simulink model "UDP_2018b"  (R2021b)
settings: Solver=FixedStepAuto  StartTime=0.0  StopTime=inf  FixedStep=0.01  RelTol=1e-3
undefined symbols (not defined in the file): Angle, Axis, magnitude, R_threshold, theta1
libraries: dspstat3 x3, dspnetwork x2, simulink_extras x1, robotcorelib x1
settings Model: Creator=OKADA  LastModifiedBy=村尾研究室
settings SolverCC: AlgebraicLoopSolver=TrustRegion
settings DataIOCC: ReturnWorkspaceOutputs=off
settings DebuggingCC: SFMachineParentedDataDiag=warning  ArithmeticOperatorsInVariantConditions=warning
settings SFSimCC: CustomCodeUndefinedFunction=UseInterfaceOnly
settings RTWCC: DLArmComputeVersion=20.02.1

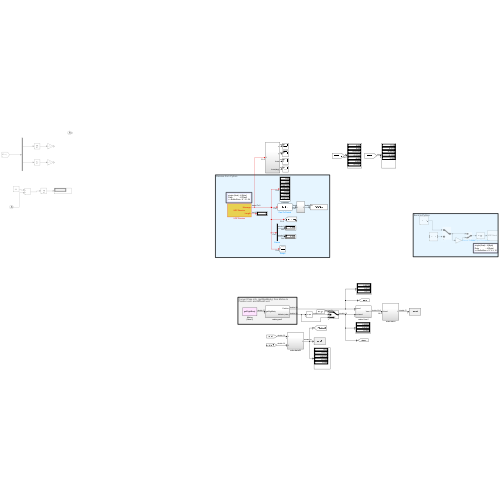
[thumbnail: Simulink's stored preview of the top-level diagram]
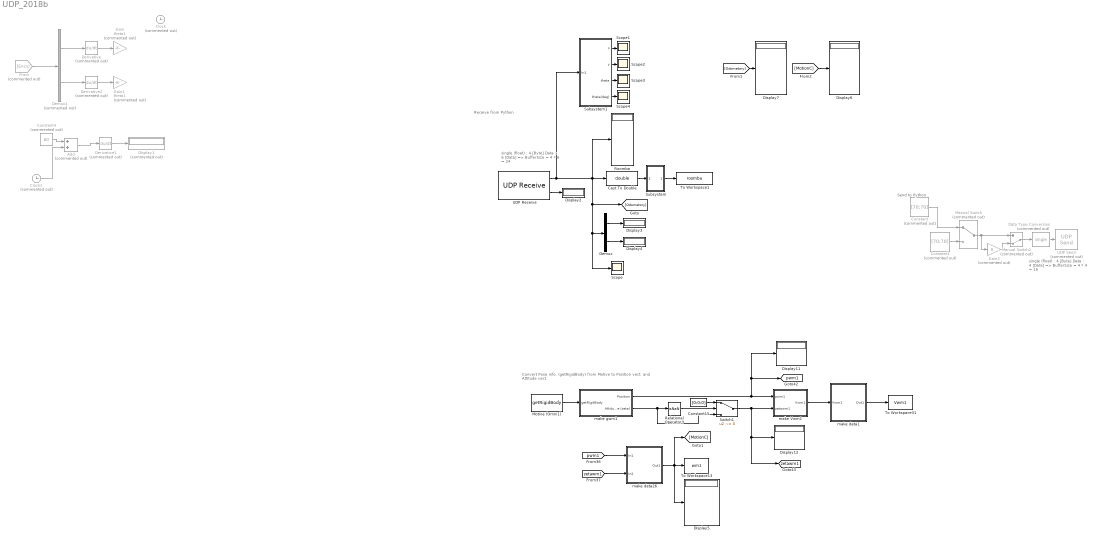
== system UDP_2018b ==
  note: Send to Python
  note: Receive from Python
  note: single (float) : 4 [Byte]
      | Data             : 6 [Data]
      | => BufferSize = 4 * 6 = 24
  note: single (float) : 4 [Byte]
      | Data             : 4 [Data]
      | => BufferSize = 4 * 4 = 16
  note: Convert Pose info. (getRigidBody) from Motive to
      | Position vect. and Attitude vect.
  Add : Sum  Commented=on
  Cast To Double : DataTypeConversion  OutDataTypeStr=double
  Clock : Clock  Commented=on
  Clock1 : Clock  Commented=on
  Constant : Constant  Commented=on  Value=[70;70]
  Constant1 : Constant  Commented=on  Value=[70;70]
  Constant15 : Constant  Value=[0;0;0]
  Constant4 : Constant  Commented=on  Value=60
  Data Type Conversion : DataTypeConversion  Commented=on  OutDataTypeStr=single
  Demux : Demux  Outputs=2
  Demux1 : Demux  Commented=on  Outputs=2
  Derivative : Derivative  Commented=on
  Derivative1 : Derivative  Commented=on
  Derivative2 : Derivative  Commented=on
  Display1 : Display  Commented=on
  Display{2..7,11..12} (8 alike) : Display
  From : From  Commented=on  GotoTag=Encs
  Gain : Gain  Commented=on  Gain=theta1
  Gain1 : Gain  Commented=on  Gain=theta1
  Gain3 : Gain  Commented=on  Gain=0
  Manual Switch : ManualSwitch  Commented=on
  Manual Switch2 : ManualSwitch  Commented=on  CurrentSetting=0
  Motive (Omni1) : M-S-Function  FunctionName=getRigidBody  Parameters=1
  Relational Operator3 : RelationalOperator  Operator=isNaN  OutDataTypeStr=boolean  RndMeth=Simplest
  Roomba : Display
  Scope{,1..4} (5 alike) : Scope
  Subsystem : Subsystem
  Subsystem1 : Subsystem
  Switch1 : Switch  Criteria=u2 ~= 0
  To Workspace1 : ToWorkspace  VariableName=roomba  SaveFormat=Structure With Time  SampleTime=-1
  To Workspace13 : ToWorkspace  VariableName=wm1  SaveFormat=Structure With Time  SampleTime=-1
  To Workspace31 : ToWorkspace  VariableName=Vwm1  SaveFormat=Structure With Time  SampleTime=-1
  UDP Receive : dspnetwork/UDP Receive  localURL='0.0.0.0'  localPort=4000  remoteURL='127.0.0.1'  remotePort=-1  recvBufferSize=28  dims=7  signalDatatype=single  isComplex=off  isVarSize=off  showBlockingTime=off  blockingTime=0  sampletime=0.01  blockPlatform=[]
  UDP Send : dspnetwork/UDP Send  Commented=on  remoteURL='127.0.0.1'  remotePort=8000  localURL='0.0.0.0'  localPortSource=Automatically determine  localPort=-1  sendBufferSize=8192  sampletime=-1  blockPlatform=[]  separateLengthPort=0
  make Vwm1 : Subsystem
  make data1 : Subsystem
  make data26 : Subsystem
  make gwm1 : Subsystem
  tag scope: pwm1=global, zetawm1=global
  wires:
  UDP Receive/2 -> Display2/1
  UDP Receive/1 -> Subsystem1/1(In1), Cast To Double/1, Roomba/1, [Odometory], Scope/1, Demux/1
  Demux/1 -> Display3/1
  Demux/2 -> Display4/1
  Manual Switch/1 -> Gain3/1, Manual Switch2/1
  Data Type Conversion/1 -> UDP Send/1
  Constant/1 -> Manual Switch/1
  Gain3/1 -> Manual Switch2/2
  Constant4/1 -> Add/1
  Add/1 -> Derivative1/1
  Clock1/1 -> Add/2
  Derivative1/1 -> Display1/1
  From/1 -> Demux1/1
  Demux1/1 -> Derivative/1
  Demux1/2 -> Derivative2/1
  Derivative/1 -> Gain/1
  Derivative2/1 -> Gain1/1
  Motive (Omni1)/1 -> make gwm1/1(getRigitBody)
  Relational Operator3/1 -> Switch1/2
  make data1/1(Out1) -> To Workspace31/1
  make gwm1/1(Position) -> make Vwm1/1(pwm1), [pwm1], Display11/1
  make data26/1(Out1) -> [MotionC], To Workspace13/1, Display5/1
  [zetawm1] -> make data26/2(In2)
  make Vwm1/1(Vwm1) -> make data1/1(Vwm1)
  [pwm1] -> make data26/1(In1)
  Switch1/1 -> make Vwm1/2(zetawm1), [zetawm1], Display12/1
  Constant15/1 -> Switch1/1
  make gwm1/2(Attitude (zeta)) -> Switch1/3, Relational Operator3/1
  Cast To Double/1 -> Subsystem/1(In1)
  Subsystem/1(Out1) -> To Workspace1/1
  Manual Switch2/1 -> Data Type Conversion/1
  Constant1/1 -> Manual Switch/2
  Subsystem1/1(x) -> Scope1/1
  Subsystem1/2(y) -> Scope2/1
  Subsystem1/3(theta) -> Scope3/1
  Subsystem1/4(theta(deg)) -> Scope4/1
  [MotionC] -> Display6/1
  [Odometory] -> Display7/1

== system UDP_2018b/Subsystem ==
  In1 : Inport
  Clock2 : Clock
  Demux3 : Demux  Outputs=7
  Mux2 : Mux  Inputs=8
  Out1 : Outport
  wires:
  Demux3/6 -> Mux2/7
  Demux3/1 -> Mux2/2
  Mux2/1 -> Out1/1
  Demux3/5 -> Mux2/6
  Demux3/4 -> Mux2/5
  Demux3/7 -> Mux2/8
  In1/1 -> Demux3/1
  Demux3/3 -> Mux2/4
  Clock2/1 -> Mux2/1
  Demux3/2 -> Mux2/3

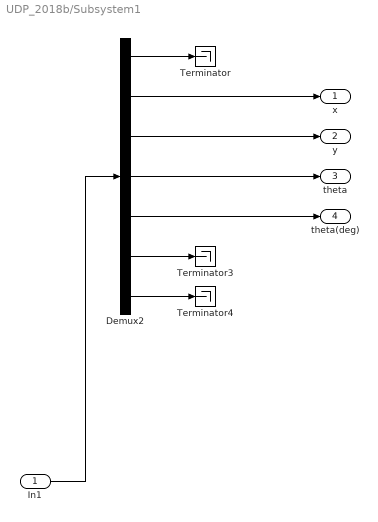
== system UDP_2018b/Subsystem1 ==
  In1 : Inport
  Demux2 : Demux  Outputs=7
  Terminator : Terminator
  Terminator3 : Terminator
  Terminator4 : Terminator
  x : Outport
  y : Outport  Port=2
  theta : Outport  Port=3
  theta(deg) : Outport  Port=4
  wires:
  Demux2/7 -> Terminator4/1
  Demux2/5 -> theta(deg)/1
  Demux2/4 -> theta/1
  Demux2/6 -> Terminator3/1
  Demux2/2 -> x/1
  In1/1 -> Demux2/1
  Demux2/1 -> Terminator/1
  Demux2/3 -> y/1

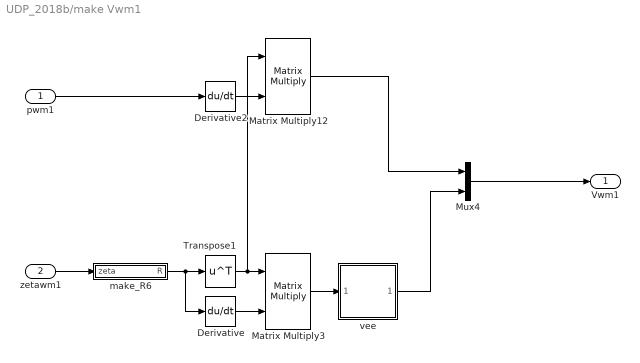
== system UDP_2018b/make Vwm1 ==
  pwm1 : Inport
  zetawm1 : Inport  Port=2
  Derivative : Derivative
  Derivative2 : Derivative
  Matrix Multiply12 : Product  Multiplication=Matrix(*)
  Matrix Multiply3 : Product  Multiplication=Matrix(*)
  Mux4 : Mux  Inputs=2
  Transpose1 : Math  Operator=transpose  SaturateOnIntegerOverflow=on
  make_R6 : Subsystem
  vee : Subsystem
  Vwm1 : Outport
  wires:
  Derivative2/1 -> Matrix Multiply12/2
  Matrix Multiply3/1 -> vee/1("[3*3]")
  Derivative/1 -> Matrix Multiply3/2
  make_R6/1(R) -> Derivative/1, Transpose1/1
  vee/1("[3*1]") -> Mux4/2
  Transpose1/1 -> Matrix Multiply12/1, Matrix Multiply3/1
  zetawm1/1 -> make_R6/1(zeta)
  Matrix Multiply12/1 -> Mux4/1
  pwm1/1 -> Derivative2/1
  Mux4/1 -> Vwm1/1

== system UDP_2018b/make data1 ==
  Vwm1 : Inport
  Clock1 : Clock
  Demux4 : Demux  Outputs=6
      settings: DisplayOption=none
  Mux2 : Mux  Inputs=7
  Out1 : Outport
  wires:
  Demux4/4 -> Mux2/5
  Demux4/5 -> Mux2/6
  Demux4/6 -> Mux2/7
  Demux4/3 -> Mux2/4
  Demux4/2 -> Mux2/3
  Demux4/1 -> Mux2/2
  Vwm1/1 -> Demux4/1
  Mux2/1 -> Out1/1
  Clock1/1 -> Mux2/1

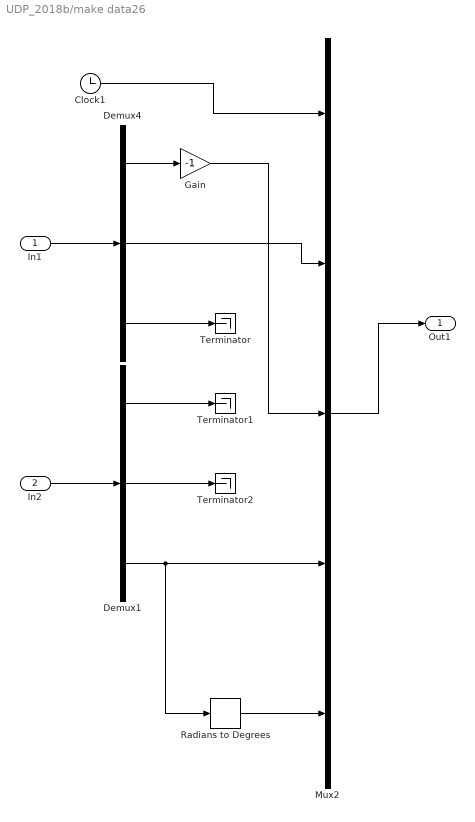
== system UDP_2018b/make data26 ==
  In1 : Inport
  In2 : Inport  Port=2
  Clock1 : Clock
  Demux1 : Demux  Outputs=3
      settings: DisplayOption=none
  Demux4 : Demux  Outputs=3
      settings: DisplayOption=none
  Gain : Gain  Gain=-1
  Mux2 : Mux  Inputs=5
  Radians to Degrees : simulink_extras/Transformations/Radians to Degrees
  Terminator : Terminator
  Terminator1 : Terminator
  Terminator2 : Terminator
  Out1 : Outport
  wires:
  Gain/1 -> Mux2/3
  Radians to Degrees/1 -> Mux2/5
  Demux1/2 -> Terminator2/1
  Demux1/1 -> Terminator1/1
  Demux4/3 -> Terminator/1
  In2/1 -> Demux1/1
  Demux1/3 -> Mux2/4, Radians to Degrees/1
  Clock1/1 -> Mux2/1
  Mux2/1 -> Out1/1
  In1/1 -> Demux4/1
  Demux4/1 -> Gain/1
  Demux4/2 -> Mux2/2

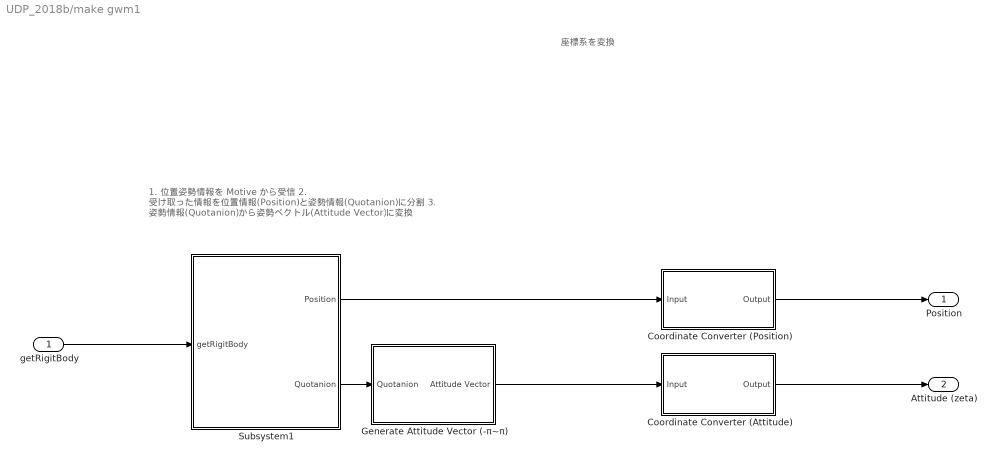
== system UDP_2018b/make gwm1 ==
  note: 1. 位置姿勢情報を Motive から受信
      | 2. 受け取った情報を位置情報(Position)と姿勢情報(Quotanion)に分割
      | 3. 姿勢情報(Quotanion)から姿勢ベクトル(Attitude Vector)に変換
  note: 座標系を変換
  getRigitBody : Inport
  Coordinate Converter (Attitude) : Subsystem
  Coordinate Converter (Position) : Subsystem
  Generate Attitude Vector (-π~π) : Subsystem
  Subsystem1 : Subsystem
  Position : Outport  VectorParamsAs1DForOutWhenUnconnected=off
  Attitude (zeta) : Outport  Port=2  VectorParamsAs1DForOutWhenUnconnected=off
  wires:
  Coordinate Converter (Attitude)/1(Output) -> Attitude (zeta)/1
  Coordinate Converter (Position)/1(Output) -> Position/1
  Subsystem1/1(Position) -> Coordinate Converter (Position)/1(Input)
  Generate Attitude Vector (-π~π)/1(Attitude Vector) -> Coordinate Converter (Attitude)/1(Input)
  getRigitBody/1 -> Subsystem1/1(getRigitBody)
  Subsystem1/2(Quotanion) -> Generate Attitude Vector (-π~π)/1(Quotanion)

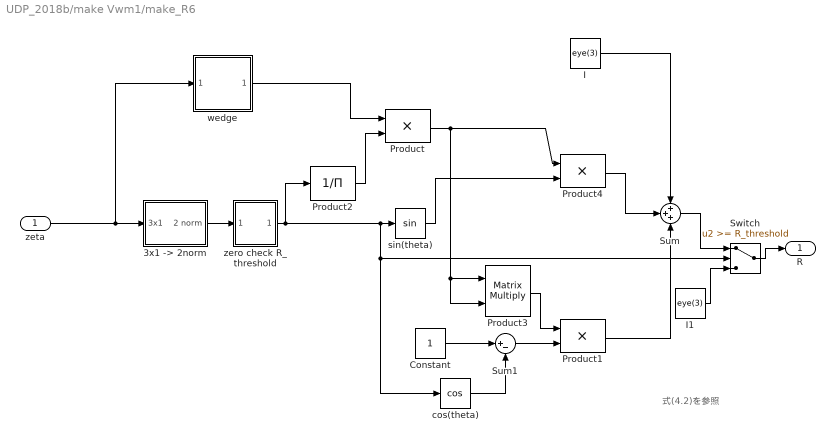
== system UDP_2018b/make Vwm1/make_R6 ==
  note: 式(4.2)を参照
  zeta : Inport
  "3x1 -> 2norm" : Subsystem
  Constant : Constant
  I : Constant  Value=eye(3)  VectorParams1D=off
  I1 : Constant  Value=eye(3)  VectorParams1D=off
  Product : Product  InputSameDT=on  SaturateOnIntegerOverflow=on  OutDataTypeStr=Inherit: Same as first input
  Product1 : Product  InputSameDT=on  SaturateOnIntegerOverflow=on  OutDataTypeStr=Inherit: Same as first input
  Product2 : Product  Inputs=/  InputSameDT=on  SaturateOnIntegerOverflow=on  OutDataTypeStr=Inherit: Same as first input
  Product3 : Product  Multiplication=Matrix(*)  InputSameDT=on  SaturateOnIntegerOverflow=on  OutDataTypeStr=Inherit: Same as first input
  Product4 : Product  InputSameDT=on  SaturateOnIntegerOverflow=on  OutDataTypeStr=Inherit: Same as first input
  Sum : Sum  Inputs=+++  InputSameDT=on  SaturateOnIntegerOverflow=on  OutDataTypeStr=Inherit: Same as first input
  Sum1 : Sum  Inputs=|+-  InputSameDT=on  SaturateOnIntegerOverflow=on  OutDataTypeStr=Inherit: Same as first input
  Switch : Switch  Threshold=R_threshold  SaturateOnIntegerOverflow=on  InputSameDT=on
  cos(theta) : Trigonometry  Operator=cos
  sin(theta) : Trigonometry
  wedge : Subsystem
  zero check R_threshold : Subsystem
  R : Outport  VectorParamsAs1DForOutWhenUnconnected=off
  wires:
  Product4/1 -> Sum/2
  Product1/1 -> Sum/3
  Sum1/1 -> Product1/2
  cos(theta)/1 -> Sum1/2
  Constant/1 -> Sum1/1
  I/1 -> Sum/1
  sin(theta)/1 -> Product4/2
  Sum/1 -> Switch/1
  I1/1 -> Switch/3
  Switch/1 -> R/1
  "3x1 -> 2norm"/1(2 norm) -> zero check R_threshold/1(In1)
  Product/1 -> Product4/1, Product3/1, Product3/2
  wedge/1("[3x3]") -> Product/1
  zero check R_threshold/1(Out1) -> Product2/1, sin(theta)/1, Switch/2, cos(theta)/1
  Product2/1 -> Product/2
  zeta/1 -> "3x1 -> 2norm"/1(3x1), wedge/1("[3x1]")
  Product3/1 -> Product1/1

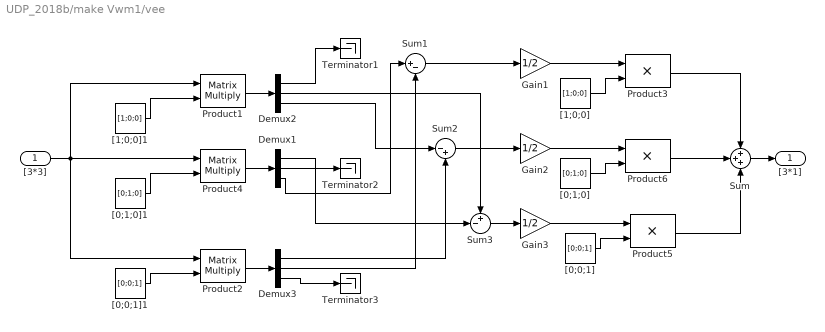
== system UDP_2018b/make Vwm1/vee ==
  "[3*3]" : Inport
  Demux1 : Demux  Outputs=3
      settings: DisplayOption=none
  Demux2 : Demux  Outputs=3
      settings: DisplayOption=none
  Demux3 : Demux  Outputs=3
      settings: DisplayOption=none
  Gain1 : Gain  Gain=1/2  SaturateOnIntegerOverflow=on  OutDataTypeStr=Inherit: Same as input  ParamDataTypeStr=Inherit: Same as input
  Gain2 : Gain  Gain=1/2  SaturateOnIntegerOverflow=on  OutDataTypeStr=Inherit: Same as input  ParamDataTypeStr=Inherit: Same as input
  Gain3 : Gain  Gain=1/2  SaturateOnIntegerOverflow=on  OutDataTypeStr=Inherit: Same as input  ParamDataTypeStr=Inherit: Same as input
  Product1 : Product  Multiplication=Matrix(*)  InputSameDT=on  SaturateOnIntegerOverflow=on  OutDataTypeStr=Inherit: Same as first input
  Product2 : Product  Multiplication=Matrix(*)  InputSameDT=on  SaturateOnIntegerOverflow=on  OutDataTypeStr=Inherit: Same as first input
  Product3 : Product  InputSameDT=on  SaturateOnIntegerOverflow=on  OutDataTypeStr=Inherit: Same as first input
  Product4 : Product  Multiplication=Matrix(*)  InputSameDT=on  SaturateOnIntegerOverflow=on  OutDataTypeStr=Inherit: Same as first input
  Product5 : Product  InputSameDT=on  SaturateOnIntegerOverflow=on  OutDataTypeStr=Inherit: Same as first input
  Product6 : Product  InputSameDT=on  SaturateOnIntegerOverflow=on  OutDataTypeStr=Inherit: Same as first input
  Sum : Sum  Inputs=+++  InputSameDT=on  SaturateOnIntegerOverflow=on  OutDataTypeStr=Inherit: Same as first input
  Sum1 : Sum  Inputs=|+-  InputSameDT=on  SaturateOnIntegerOverflow=on  OutDataTypeStr=Inherit: Same as first input
  Sum2 : Sum  Inputs=|-+  InputSameDT=on  SaturateOnIntegerOverflow=on  OutDataTypeStr=Inherit: Same as first input
  Sum3 : Sum  Inputs=+-|  InputSameDT=on  SaturateOnIntegerOverflow=on  OutDataTypeStr=Inherit: Same as first input
  Terminator1 : Terminator
  Terminator2 : Terminator
  Terminator3 : Terminator
  "[0;0;1]" : Constant  Value=[0;0;1]  VectorParams1D=off
  "[0;0;1]1" : Constant  Value=[0;0;1]  VectorParams1D=off
  "[0;1;0]" : Constant  Value=[0;1;0]  VectorParams1D=off
  "[0;1;0]1" : Constant  Value=[0;1;0]  VectorParams1D=off
  "[1;0;0]" : Constant  Value=[1;0;0]  VectorParams1D=off
  "[1;0;0]1" : Constant  Value=[1;0;0]  VectorParams1D=off
  "[3*1]" : Outport  VectorParamsAs1DForOutWhenUnconnected=off
  wires:
  "[3*3]"/1 -> Product2/1, Product1/1, Product4/1
  "[0;1;0]1"/1 -> Product4/2
  Product4/1 -> Demux1/1
  Demux1/2 -> Terminator2/1
  Demux1/3 -> Sum1/1
  "[1;0;0]1"/1 -> Product1/2
  Product1/1 -> Demux2/1
  Demux2/1 -> Terminator1/1
  "[0;0;1]1"/1 -> Product2/2
  Product2/1 -> Demux3/1
  Demux3/3 -> Terminator3/1
  Demux3/1 -> Sum2/2
  "[1;0;0]"/1 -> Product3/2
  "[0;1;0]"/1 -> Product6/2
  "[0;0;1]"/1 -> Product5/2
  Product6/1 -> Sum/2
  Product5/1 -> Sum/3
  Product3/1 -> Sum/1
  Sum/1 -> "[3*1]"/1
  Sum1/1 -> Gain1/1
  Gain1/1 -> Product3/1
  Demux3/2 -> Sum1/2
  Gain2/1 -> Product6/1
  Gain3/1 -> Product5/1
  Demux2/3 -> Sum2/1
  Sum2/1 -> Gain2/1
  Sum3/1 -> Gain3/1
  Demux2/2 -> Sum3/1
  Demux1/1 -> Sum3/2

== system UDP_2018b/make gwm1/Coordinate Converter (Attitude) ==
  Input : Inport
  Demux : Demux  Outputs=3
  Mux : Mux  Inputs=3
  Output : Outport  VectorParamsAs1DForOutWhenUnconnected=off
  wires:
  Demux/3 -> Mux/1
  Demux/1 -> Mux/2
  Demux/2 -> Mux/3
  Mux/1 -> Output/1
  Input/1 -> Demux/1

== system UDP_2018b/make gwm1/Coordinate Converter (Position) ==
  Input : Inport
  Demux : Demux  Outputs=3
  Mux : Mux  Inputs=3
  Output : Outport  VectorParamsAs1DForOutWhenUnconnected=off
  wires:
  Demux/3 -> Mux/1
  Demux/1 -> Mux/2
  Demux/2 -> Mux/3
  Mux/1 -> Output/1
  Input/1 -> Demux/1

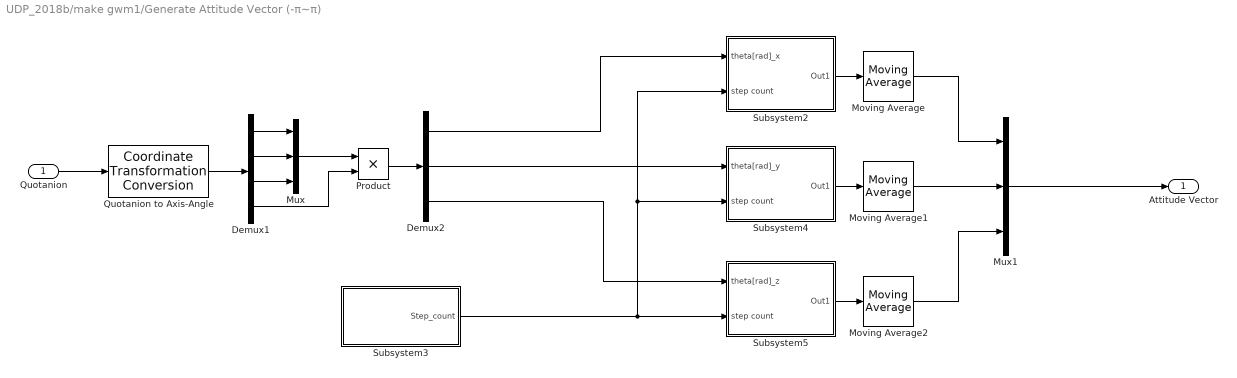
== system UDP_2018b/make gwm1/Generate Attitude Vector (-π~π) ==
  Quotanion : Inport
  Demux1 : Demux
  Demux2 : Demux  Outputs=3
  Moving Average : dspstat3/Moving Average  Method=Sliding window  ForgettingFactorPort=off  SpecifyWindowLength=on  WindowLength=10  ForgettingFactor=0.9  SimulateUsing=Code generation
  Moving Average1 : dspstat3/Moving Average  Method=Sliding window  ForgettingFactorPort=off  SpecifyWindowLength=on  WindowLength=10  ForgettingFactor=0.9  SimulateUsing=Code generation
  Moving Average2 : dspstat3/Moving Average  Method=Sliding window  ForgettingFactorPort=off  SpecifyWindowLength=on  WindowLength=10  ForgettingFactor=0.9  SimulateUsing=Code generation
  Mux : Mux  Inputs=3
  Mux1 : Mux  Inputs=3
  Product : Product
  Quotanion to Axis-Angle : robotcorelib/Coordinate Transformation Conversion  InputRepresentation=Quaternion  InputEulerSequence=ZYX  ShowTrVecInputPort=on  OutputRepresentation=Axis-Angle  OutputEulerSequence=ZYX  ShowTrVecOutputPort=on  SimulateUsing=Interpreted execution
      settings: SourceProductBaseCode=NV,RO,RR,UV
  Subsystem2 : Subsystem
  Subsystem3 : Subsystem
  Subsystem4 : Subsystem
  Subsystem5 : Subsystem
  Attitude Vector : Outport  VectorParamsAs1DForOutWhenUnconnected=off
  wires:
  Quotanion/1 -> Quotanion to Axis-Angle/1
  Mux1/1 -> Attitude Vector/1
  Moving Average2/1 -> Mux1/3
  Moving Average1/1 -> Mux1/2
  Product/1 -> Demux2/1
  Mux/1 -> Product/1
  Demux1/4 -> Product/2
  Demux2/3 -> Subsystem5/1(theta[rad]_z)
  Demux2/2 -> Subsystem4/1(theta[rad]_y)
  Demux1/3 -> Mux/3
  Demux1/1 -> Mux/1
  Demux1/2 -> Mux/2
  Subsystem2/1(Out1) -> Moving Average/1
  Demux2/1 -> Subsystem2/1(theta[rad]_x)
  Quotanion to Axis-Angle/1 -> Demux1/1
  Subsystem3/1(Step_count) -> Subsystem5/2(step count), Subsystem4/2(step count), Subsystem2/2(step count)
  Subsystem5/1(Out1) -> Moving Average2/1
  Subsystem4/1(Out1) -> Moving Average1/1
  Moving Average/1 -> Mux1/1

== system UDP_2018b/make gwm1/Subsystem1 ==
  getRigitBody : Inport
  Demux : Demux  Outputs=7
  Mux1 : Mux
  Mux6 : Mux  Inputs=3
  Position : Outport  VectorParamsAs1DForOutWhenUnconnected=off
  Quotanion : Outport  Port=2  VectorParamsAs1DForOutWhenUnconnected=off
  wires:
  Demux/1 -> Mux6/1
  Demux/3 -> Mux6/3
  Demux/2 -> Mux6/2
  Mux1/1 -> Quotanion/1
  Demux/7 -> Mux1/4
  Demux/6 -> Mux1/3
  Demux/5 -> Mux1/2
  Demux/4 -> Mux1/1
  getRigitBody/1 -> Demux/1
  Mux6/1 -> Position/1

== system UDP_2018b/make Vwm1/make_R6/3x1 -> 2norm ==
  3x1 : Inport
  Demux : Demux  Outputs=3
      settings: DisplayOption=none
  Math Function : Math  Operator=magnitude^2  SignedPower=on  SaturateOnIntegerOverflow=on
  Math Function1 : Math  Operator=sqrt  SignedPower=on  SaturateOnIntegerOverflow=on
  Sum : Sum  Inputs=+++  InputSameDT=on  SaturateOnIntegerOverflow=on  OutDataTypeStr=Inherit: Same as first input
  2 norm : Outport  VectorParamsAs1DForOutWhenUnconnected=off
  wires:
  3x1/1 -> Math Function/1
  Math Function1/1 -> 2 norm/1
  Sum/1 -> Math Function1/1
  Demux/1 -> Sum/1
  Demux/2 -> Sum/2
  Demux/3 -> Sum/3
  Math Function/1 -> Demux/1

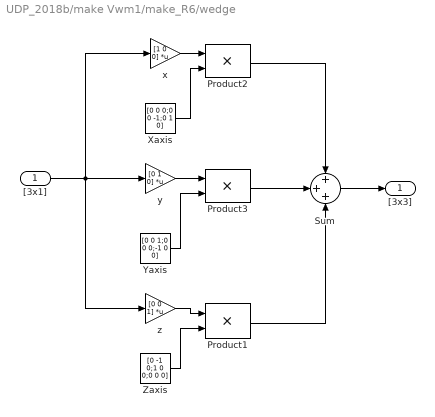
== system UDP_2018b/make Vwm1/make_R6/wedge ==
  "[3x1]" : Inport
  Product1 : Product  InputSameDT=on  SaturateOnIntegerOverflow=on  OutDataTypeStr=Inherit: Same as first input
  Product2 : Product  InputSameDT=on  SaturateOnIntegerOverflow=on  OutDataTypeStr=Inherit: Same as first input
  Product3 : Product  InputSameDT=on  SaturateOnIntegerOverflow=on  OutDataTypeStr=Inherit: Same as first input
  Sum : Sum  Inputs=+++  InputSameDT=on  SaturateOnIntegerOverflow=on  OutDataTypeStr=Inherit: Same as first input
  Xaxis : Constant  Value=[0 0 0;0 0 -1;0 1 0]  VectorParams1D=off
  Yaxis : Constant  Value=[0 0 1;0 0 0;-1 0 0]  VectorParams1D=off
  Zaxis : Constant  Value=[0 -1 0;1 0 0;0 0 0]  VectorParams1D=off
  x : Gain  Gain=[1 0 0]  Multiplication=Matrix(K*u)  SaturateOnIntegerOverflow=on  OutDataTypeStr=Inherit: Same as input  ParamDataTypeStr=Inherit: Same as input
  y : Gain  Gain=[0 1 0]  Multiplication=Matrix(K*u)  SaturateOnIntegerOverflow=on  OutDataTypeStr=Inherit: Same as input  ParamDataTypeStr=Inherit: Same as input
  z : Gain  Gain=[0 0 1]  Multiplication=Matrix(K*u)  SaturateOnIntegerOverflow=on  OutDataTypeStr=Inherit: Same as input  ParamDataTypeStr=Inherit: Same as input
  "[3x3]" : Outport  VectorParamsAs1DForOutWhenUnconnected=off
  wires:
  Zaxis/1 -> Product1/2
  z/1 -> Product1/1
  Xaxis/1 -> Product2/2
  x/1 -> Product2/1
  Yaxis/1 -> Product3/2
  y/1 -> Product3/1
  "[3x1]"/1 -> y/1, x/1, z/1
  Product3/1 -> Sum/2
  Product2/1 -> Sum/1
  Product1/1 -> Sum/3
  Sum/1 -> "[3x3]"/1

== system UDP_2018b/make Vwm1/make_R6/zero check R_threshold ==
  In1 : Inport
  Switch : Switch  Threshold=R_threshold  SaturateOnIntegerOverflow=on  InputSameDT=on
  norm_xi : Constant  Value=R_threshold  VectorParams1D=off
  Out1 : Outport  VectorParamsAs1DForOutWhenUnconnected=off
  wires:
  norm_xi/1 -> Switch/3
  In1/1 -> Switch/1, Switch/2
  Switch/1 -> Out1/1

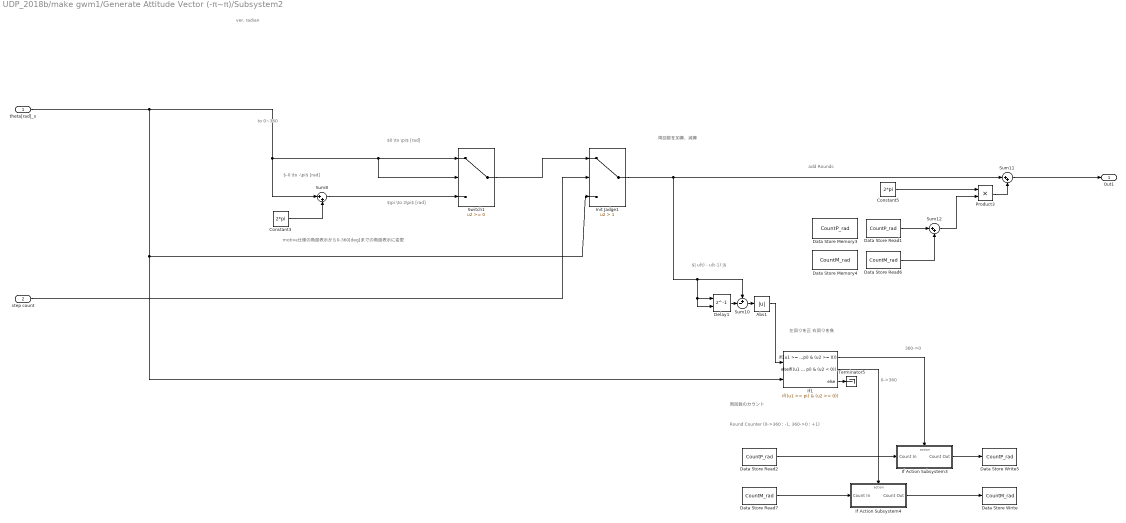
== system UDP_2018b/make gwm1/Generate Attitude Vector (-π~π)/Subsystem2 ==
  note: $0 \to \pi$ [rad]
  note: ver. radian
  note: 周回数を加算、減算
  note: motive仕様の角度表示から0-360[deg]までの角度表示に変更
  note: to 0~360
  note: 360->0
  note: add Rounds
  note: $-0 \to -\pi$ [rad]
  note: $\pi \to 2\pi$ [rad]
  note: 0->360
  note: $| u(t) - u(t-1) |$
  note: Round Counter (0->360 : -1, 360->0 : +1)
  note: 左回りを正
      | 右回りを負
  note: 周回数のカウント
  theta[rad]_x : Inport
  step count : Inport  Port=2
  Abs1 : Abs
  Constant3 : Constant  Value=2*pi
  Constant5 : Constant  Value=2*pi
  Data Store Memory3 : DataStoreMemory  DataStoreName=CountP_rad  ReadBeforeWriteMsg=warning  WriteAfterWriteMsg=warning  WriteAfterReadMsg=warning  ShowAdditionalParam=off
  Data Store Memory4 : DataStoreMemory  DataStoreName=CountM_rad  ReadBeforeWriteMsg=warning  WriteAfterWriteMsg=warning  WriteAfterReadMsg=warning  ShowAdditionalParam=off
  Data Store Read1 : DataStoreRead  DataStoreName=CountP_rad  IndexOptions=Index vector (dialog)  Indices=1  OutputSizes=1
  Data Store Read2 : DataStoreRead  DataStoreName=CountP_rad  IndexOptions=Index vector (dialog)  Indices=1  OutputSizes=1
  Data Store Read6 : DataStoreRead  DataStoreName=CountM_rad  IndexOptions=Index vector (dialog)  Indices=1  OutputSizes=1
  Data Store Read7 : DataStoreRead  DataStoreName=CountM_rad  IndexOptions=Index vector (dialog)  Indices=1  OutputSizes=1
  Data Store Write : DataStoreWrite  DataStoreName=CountM_rad  IndexOptions=Index vector (dialog)  Indices=1  OutputSizes=1
  Data Store Write5 : DataStoreWrite  DataStoreName=CountP_rad  IndexOptions=Index vector (dialog)  Indices=1  OutputSizes=1
  Delay1 : Delay  DelayLength=1  InitialConditionSource=Input port  InitialCondition=0
      settings: InputPortMap=u0,p4
  If Action Subsystem3 : Subsystem  TreatAsAtomicUnit=on
  If Action Subsystem4 : Subsystem  TreatAsAtomicUnit=on
  If1 : If  NumInputs=2  IfExpression=(u1 >= pi) & (u2 >= 0)  ElseIfExpressions=(u1 >= pi) & (u2 < 0)
  Init Jadge1 : Switch  Criteria=u2 > Threshold  Threshold=1
  Product3 : Product
  Sum10 : Sum  Inputs=+-|
  Sum11 : Sum  Inputs=|++
  Sum12 : Sum  Inputs=|++
  Sum8 : Sum  Inputs=|++
  Switch1 : Switch
  Terminator5 : Terminator
  Out1 : Outport  VectorParamsAs1DForOutWhenUnconnected=off
  wires:
  step count/1 -> Init Jadge1/2
  Sum11/1 -> Out1/1
  Data Store Read6/1 -> Sum12/2
  Data Store Read2/1 -> If Action Subsystem3/1(Count In)
  If Action Subsystem3/1(Count Out) -> Data Store Write5/1
  If1/3 -> Terminator5/1
  Constant5/1 -> Product3/1
  Sum12/1 -> Product3/2
  If1/2 -> If Action Subsystem4/Action
  If Action Subsystem4/1(Count Out) -> Data Store Write/1
  Delay1/1 -> Sum10/2
  Product3/1 -> Sum11/2
  Init Jadge1/1 -> Sum11/1, Sum10/1, Delay1/1, Delay1/2
  theta[rad]_x/1 -> Sum8/1, Switch1/2, Switch1/1, Init Jadge1/3, If1/2
  Sum8/1 -> Switch1/3
  Constant3/1 -> Sum8/2
  Switch1/1 -> Init Jadge1/1
  Data Store Read7/1 -> If Action Subsystem4/1(Count In)
  Data Store Read1/1 -> Sum12/1
  Abs1/1 -> If1/1
  Sum10/1 -> Abs1/1
  If1/1 -> If Action Subsystem3/Action

== system UDP_2018b/make gwm1/Generate Attitude Vector (-π~π)/Subsystem3 ==
  Constant2 : Constant
  Constant4 : Constant
  Delay : Delay  DelayLength=1  InitialCondition=0
  Sum7 : Sum  Inputs=|-+
  Sum9 : Sum  Inputs=++|
  Step_count : Outport  VectorParamsAs1DForOutWhenUnconnected=off
  wires:
  Delay/1 -> Sum9/1
  Sum7/1 -> Step_count/1
  Constant2/1 -> Sum7/1
  Sum9/1 -> Delay/1, Sum7/2
  Constant4/1 -> Sum9/2

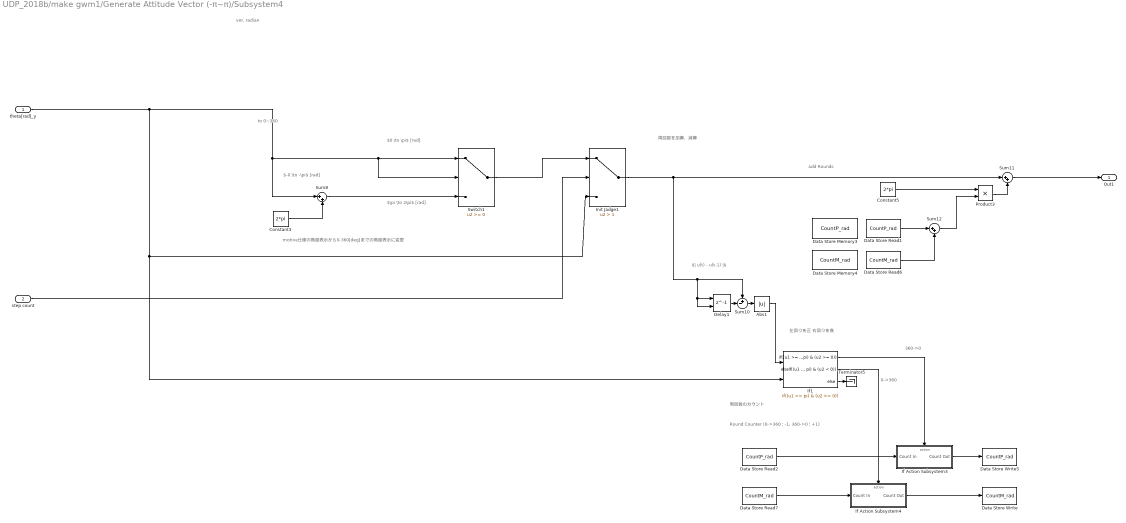
== system UDP_2018b/make gwm1/Generate Attitude Vector (-π~π)/Subsystem4 ==
  note: $0 \to \pi$ [rad]
  note: ver. radian
  note: 周回数を加算、減算
  note: motive仕様の角度表示から0-360[deg]までの角度表示に変更
  note: to 0~360
  note: 360->0
  note: add Rounds
  note: $-0 \to -\pi$ [rad]
  note: $\pi \to 2\pi$ [rad]
  note: 0->360
  note: $| u(t) - u(t-1) |$
  note: Round Counter (0->360 : -1, 360->0 : +1)
  note: 左回りを正
      | 右回りを負
  note: 周回数のカウント
  theta[rad]_y : Inport
  step count : Inport  Port=2
  Abs1 : Abs
  Constant3 : Constant  Value=2*pi
  Constant5 : Constant  Value=2*pi
  Data Store Memory3 : DataStoreMemory  DataStoreName=CountP_rad  ReadBeforeWriteMsg=warning  WriteAfterWriteMsg=warning  WriteAfterReadMsg=warning  ShowAdditionalParam=off
  Data Store Memory4 : DataStoreMemory  DataStoreName=CountM_rad  ReadBeforeWriteMsg=warning  WriteAfterWriteMsg=warning  WriteAfterReadMsg=warning  ShowAdditionalParam=off
  Data Store Read1 : DataStoreRead  DataStoreName=CountP_rad  IndexOptions=Index vector (dialog)  Indices=1  OutputSizes=1
  Data Store Read2 : DataStoreRead  DataStoreName=CountP_rad  IndexOptions=Index vector (dialog)  Indices=1  OutputSizes=1
  Data Store Read6 : DataStoreRead  DataStoreName=CountM_rad  IndexOptions=Index vector (dialog)  Indices=1  OutputSizes=1
  Data Store Read7 : DataStoreRead  DataStoreName=CountM_rad  IndexOptions=Index vector (dialog)  Indices=1  OutputSizes=1
  Data Store Write : DataStoreWrite  DataStoreName=CountM_rad  IndexOptions=Index vector (dialog)  Indices=1  OutputSizes=1
  Data Store Write5 : DataStoreWrite  DataStoreName=CountP_rad  IndexOptions=Index vector (dialog)  Indices=1  OutputSizes=1
  Delay1 : Delay  DelayLength=1  InitialConditionSource=Input port  InitialCondition=0
      settings: InputPortMap=u0,p4
  If Action Subsystem3 : Subsystem  TreatAsAtomicUnit=on
  If Action Subsystem4 : Subsystem  TreatAsAtomicUnit=on
  If1 : If  NumInputs=2  IfExpression=(u1 >= pi) & (u2 >= 0)  ElseIfExpressions=(u1 >= pi) & (u2 < 0)
  Init Jadge1 : Switch  Criteria=u2 > Threshold  Threshold=1
  Product3 : Product
  Sum10 : Sum  Inputs=+-|
  Sum11 : Sum  Inputs=|++
  Sum12 : Sum  Inputs=|++
  Sum8 : Sum  Inputs=|++
  Switch1 : Switch
  Terminator5 : Terminator
  Out1 : Outport  VectorParamsAs1DForOutWhenUnconnected=off
  wires:
  step count/1 -> Init Jadge1/2
  Sum11/1 -> Out1/1
  Data Store Read6/1 -> Sum12/2
  Data Store Read2/1 -> If Action Subsystem3/1(Count In)
  If Action Subsystem3/1(Count Out) -> Data Store Write5/1
  If1/3 -> Terminator5/1
  Constant5/1 -> Product3/1
  Sum12/1 -> Product3/2
  If1/2 -> If Action Subsystem4/Action
  If Action Subsystem4/1(Count Out) -> Data Store Write/1
  Delay1/1 -> Sum10/2
  Product3/1 -> Sum11/2
  Init Jadge1/1 -> Sum11/1, Sum10/1, Delay1/1, Delay1/2
  theta[rad]_y/1 -> Sum8/1, Switch1/2, Switch1/1, Init Jadge1/3, If1/2
  Sum8/1 -> Switch1/3
  Constant3/1 -> Sum8/2
  Switch1/1 -> Init Jadge1/1
  Data Store Read7/1 -> If Action Subsystem4/1(Count In)
  Data Store Read1/1 -> Sum12/1
  Abs1/1 -> If1/1
  Sum10/1 -> Abs1/1
  If1/1 -> If Action Subsystem3/Action

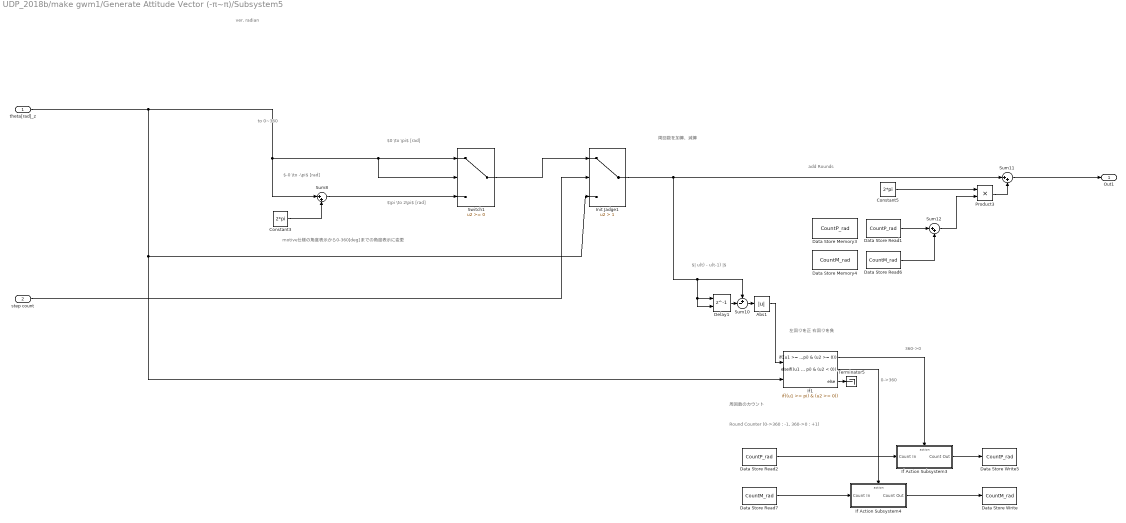
== system UDP_2018b/make gwm1/Generate Attitude Vector (-π~π)/Subsystem5 ==
  note: $0 \to \pi$ [rad]
  note: ver. radian
  note: 周回数を加算、減算
  note: motive仕様の角度表示から0-360[deg]までの角度表示に変更
  note: to 0~360
  note: 360->0
  note: add Rounds
  note: $-0 \to -\pi$ [rad]
  note: $\pi \to 2\pi$ [rad]
  note: 0->360
  note: $| u(t) - u(t-1) |$
  note: Round Counter (0->360 : -1, 360->0 : +1)
  note: 左回りを正
      | 右回りを負
  note: 周回数のカウント
  theta[rad]_z : Inport
  step count : Inport  Port=2
  Abs1 : Abs
  Constant3 : Constant  Value=2*pi
  Constant5 : Constant  Value=2*pi
  Data Store Memory3 : DataStoreMemory  DataStoreName=CountP_rad  ReadBeforeWriteMsg=warning  WriteAfterWriteMsg=warning  WriteAfterReadMsg=warning  ShowAdditionalParam=off
  Data Store Memory4 : DataStoreMemory  DataStoreName=CountM_rad  ReadBeforeWriteMsg=warning  WriteAfterWriteMsg=warning  WriteAfterReadMsg=warning  ShowAdditionalParam=off
  Data Store Read1 : DataStoreRead  DataStoreName=CountP_rad  IndexOptions=Index vector (dialog)  Indices=1  OutputSizes=1
  Data Store Read2 : DataStoreRead  DataStoreName=CountP_rad  IndexOptions=Index vector (dialog)  Indices=1  OutputSizes=1
  Data Store Read6 : DataStoreRead  DataStoreName=CountM_rad  IndexOptions=Index vector (dialog)  Indices=1  OutputSizes=1
  Data Store Read7 : DataStoreRead  DataStoreName=CountM_rad  IndexOptions=Index vector (dialog)  Indices=1  OutputSizes=1
  Data Store Write : DataStoreWrite  DataStoreName=CountM_rad  IndexOptions=Index vector (dialog)  Indices=1  OutputSizes=1
  Data Store Write5 : DataStoreWrite  DataStoreName=CountP_rad  IndexOptions=Index vector (dialog)  Indices=1  OutputSizes=1
  Delay1 : Delay  DelayLength=1  InitialConditionSource=Input port  InitialCondition=0
      settings: InputPortMap=u0,p4
  If Action Subsystem3 : Subsystem  TreatAsAtomicUnit=on
  If Action Subsystem4 : Subsystem  TreatAsAtomicUnit=on
  If1 : If  NumInputs=2  IfExpression=(u1 >= pi) & (u2 >= 0)  ElseIfExpressions=(u1 >= pi) & (u2 < 0)
  Init Jadge1 : Switch  Criteria=u2 > Threshold  Threshold=1
  Product3 : Product
  Sum10 : Sum  Inputs=+-|
  Sum11 : Sum  Inputs=|++
  Sum12 : Sum  Inputs=|++
  Sum8 : Sum  Inputs=|++
  Switch1 : Switch
  Terminator5 : Terminator
  Out1 : Outport  VectorParamsAs1DForOutWhenUnconnected=off
  wires:
  step count/1 -> Init Jadge1/2
  Sum11/1 -> Out1/1
  Data Store Read6/1 -> Sum12/2
  Data Store Read2/1 -> If Action Subsystem3/1(Count In)
  If Action Subsystem3/1(Count Out) -> Data Store Write5/1
  If1/3 -> Terminator5/1
  Constant5/1 -> Product3/1
  Sum12/1 -> Product3/2
  If1/2 -> If Action Subsystem4/Action
  If Action Subsystem4/1(Count Out) -> Data Store Write/1
  Delay1/1 -> Sum10/2
  Product3/1 -> Sum11/2
  Init Jadge1/1 -> Sum11/1, Sum10/1, Delay1/1, Delay1/2
  theta[rad]_z/1 -> Sum8/1, Switch1/2, Switch1/1, Init Jadge1/3, If1/2
  Sum8/1 -> Switch1/3
  Constant3/1 -> Sum8/2
  Switch1/1 -> Init Jadge1/1
  Data Store Read7/1 -> If Action Subsystem4/1(Count In)
  Data Store Read1/1 -> Sum12/1
  Abs1/1 -> If1/1
  Sum10/1 -> Abs1/1
  If1/1 -> If Action Subsystem3/Action

== system UDP_2018b/make gwm1/Generate Attitude Vector (-π~π)/Subsystem2/If Action Subsystem3 ==
  Count In : Inport
  Action Port : ActionPort  ActionPortLabel=if((u1 >= pi) & (u2 >= 0))
  Constant : Constant
  Sum : Sum  Inputs=|++
  Count Out : Outport  VectorParamsAs1DForOutWhenUnconnected=off
  wires:
  Count In/1 -> Sum/1
  Constant/1 -> Sum/2
  Sum/1 -> Count Out/1

== system UDP_2018b/make gwm1/Generate Attitude Vector (-π~π)/Subsystem2/If Action Subsystem4 ==
  Count In : Inport
  Action Port : ActionPort  ActionPortLabel=elseif((u1 >= pi) & (u2 < 0))
  Constant : Constant
  Sum : Sum  Inputs=|+-
  Count Out : Outport  VectorParamsAs1DForOutWhenUnconnected=off
  wires:
  Sum/1 -> Count Out/1
  Constant/1 -> Sum/2
  Count In/1 -> Sum/1

== system UDP_2018b/make gwm1/Generate Attitude Vector (-π~π)/Subsystem4/If Action Subsystem3 ==
  Count In : Inport
  Action Port : ActionPort  ActionPortLabel=if((u1 >= pi) & (u2 >= 0))
  Constant : Constant
  Sum : Sum  Inputs=|++
  Count Out : Outport  VectorParamsAs1DForOutWhenUnconnected=off
  wires:
  Count In/1 -> Sum/1
  Constant/1 -> Sum/2
  Sum/1 -> Count Out/1

== system UDP_2018b/make gwm1/Generate Attitude Vector (-π~π)/Subsystem4/If Action Subsystem4 ==
  Count In : Inport
  Action Port : ActionPort  ActionPortLabel=elseif((u1 >= pi) & (u2 < 0))
  Constant : Constant
  Sum : Sum  Inputs=|+-
  Count Out : Outport  VectorParamsAs1DForOutWhenUnconnected=off
  wires:
  Sum/1 -> Count Out/1
  Constant/1 -> Sum/2
  Count In/1 -> Sum/1

== system UDP_2018b/make gwm1/Generate Attitude Vector (-π~π)/Subsystem5/If Action Subsystem3 ==
  Count In : Inport
  Action Port : ActionPort  ActionPortLabel=if((u1 >= pi) & (u2 >= 0))
  Constant : Constant
  Sum : Sum  Inputs=|++
  Count Out : Outport  VectorParamsAs1DForOutWhenUnconnected=off
  wires:
  Count In/1 -> Sum/1
  Constant/1 -> Sum/2
  Sum/1 -> Count Out/1

== system UDP_2018b/make gwm1/Generate Attitude Vector (-π~π)/Subsystem5/If Action Subsystem4 ==
  Count In : Inport
  Action Port : ActionPort  ActionPortLabel=elseif((u1 >= pi) & (u2 < 0))
  Constant : Constant
  Sum : Sum  Inputs=|+-
  Count Out : Outport  VectorParamsAs1DForOutWhenUnconnected=off
  wires:
  Sum/1 -> Count Out/1
  Constant/1 -> Sum/2
  Count In/1 -> Sum/1
